simulink model "FOC_IF"  (R2023b)
settings: Solver=FixedStepDiscrete  StartTime=0.0  StopTime=1  FixedStep=0.000001  RelTol=1e-3
undefined symbols (not defined in the file): Pn, Udc
libraries: mcbplantlib x1, autolibpmsmexterior x1, simulink x1
settings Model: DataDictionary=SVPWM.sldd  Creator=18575  LastModifiedBy=Administrator

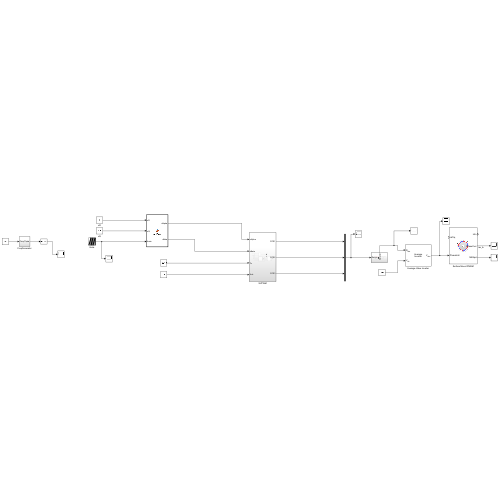
[thumbnail: Simulink's stored preview of the top-level diagram]
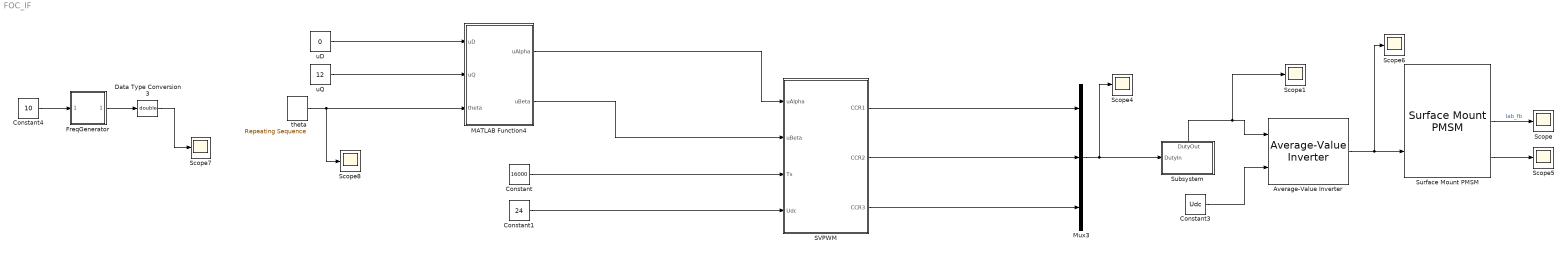
== system FOC_IF ==
  Average-Value Inverter : mcbplantlib/Average-Value Inverter
  Constant : Constant  Value=16000
  Constant1 : Constant  Value=24
  Constant3 : Constant  Value=Udc
  Constant4 : Constant  Value=10  OutDataTypeStr=single
  Data Type Conversion3 : DataTypeConversion  OutDataTypeStr=double  SaturateOnIntegerOverflow=off  RndMeth=Floor
  FreqGenerator : Subsystem
  MATLAB Function4 : MATLAB Function  TreatAsAtomicUnit=on
  Mux3 : Mux  Inputs=3
  SVPWM : Subsystem
  Scope{,1,4..8} (7 alike) : Scope
  Subsystem : Subsystem
      settings: PortSchema="{\"entries\":[{\"content\":{\"sides\":[{\"content\":{\"connectorIds\":[\"In1\"]},\"type\":\"ConnectorPlacement.EquallySpacedRectSide\",\"uuid\":\"8ccc51de-fa2a-4900-80a3-4cdf9aa76f01\"},{\"content\":{\"side\":\"RIGHT\"},\"type\":\"ConnectorPlacement.EquallySpacedRectSide\",\"uuid\":\"32c06e0d-3f1d-4948-af96-e310e54308a0\"},{\"content\":{\"connectorIds\":[\"Out1\"],\"side\":\"TOP\"},\"type\":\"ConnectorPlacement.EquallySpacedRectSide\",\"uuid\":\"a9066067-2c54-42a8-b4d7-fb86ac71b860\"}]},\"type\":\"ConnectorPlacement.EquallySpacedConnector\",\"uuid\":\"e4576975-acad-4e16-822f-2c2e7f23d7a7\"}],\"packageUris\":[\"http://schema.mathworks.com/mf0/Connector/R2020b\"],\"version\":\"1.0\"}"
  Surface Mount PMSM : autolibpmsmexterior/Surface Mount PMSM  port_config=Torque  sim_type=Discrete  Ts=1e-4  P=Pn  Rs=Rs  Ldq_=L  KConstText=Permanent flux linkage constant (lambda_pm):  lambda_pm=flux  Ke=0.0059268  Kt=0.061  mechanical=[75e-6, 8e-5, 0]  idq0=[0 0]  theta_init=4/5  omega_init=0  KConst=flux  lambda_pm_calc=flux  RefBlkName='autolibpmsmexterior/Surface Mount PMSM'  aMode=5  Ldq="[0.0017      0.0017]"
  "theta " : simulink/Sources/Repeating Sequence  rep_seq_t=[0 0.5]  rep_seq_y=[0 2*pi]
  uD : Constant  Value=0
  uQ : Constant  Value=12
  wires:
  uQ/1 -> MATLAB Function4/2(uQ)
  uD/1 -> MATLAB Function4/1(uD)
  Mux3/1 -> Scope4/1, Subsystem/1(DutyIn)
  Subsystem/1(DutyOut) -> Scope1/1, Average-Value Inverter/1
  Constant3/1 -> Average-Value Inverter/2
  Average-Value Inverter/1 -> Scope6/1, Surface Mount PMSM/2
  Surface Mount PMSM/2 -> Scope/1  "Iab_fb"
  Surface Mount PMSM/3 -> Scope5/1
  FreqGenerator/1(Theta) -> Data Type Conversion3/1
  Constant4/1 -> FreqGenerator/1(Freq)
  Data Type Conversion3/1 -> Scope7/1
  "theta "/1 -> Scope8/1, MATLAB Function4/3(theta)
  MATLAB Function4/1(uAlpha) -> SVPWM/1(uAlpha)
  MATLAB Function4/2(uBeta) -> SVPWM/2(uBeta)
  Constant/1 -> SVPWM/3(Ts)
  Constant1/1 -> SVPWM/4(Udc)
  SVPWM/1(CCR1) -> Mux3/1
  SVPWM/2(CCR2) -> Mux3/2
  SVPWM/3(CCR3) -> Mux3/3

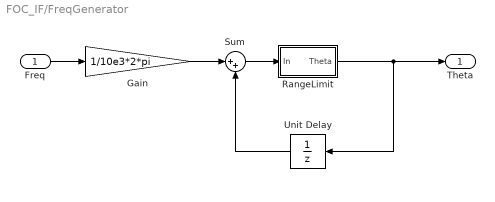
== system FOC_IF/FreqGenerator ==
  Freq : Inport
  Gain : Gain  Gain=1/10e3*2*pi  OutDataTypeStr=single
  RangeLimit : Subsystem
  Sum : Sum  Inputs=|++  OutDataTypeStr=Inherit: Same as first input
  Unit Delay : UnitDelay  SampleTime=-1  HasFrameUpgradeWarning=on
  Theta : Outport
  wires:
  Freq/1 -> Gain/1
  RangeLimit/1(Theta) -> Theta/1, Unit Delay/1
  Gain/1 -> Sum/1
  Sum/1 -> RangeLimit/1(In)
  Unit Delay/1 -> Sum/2

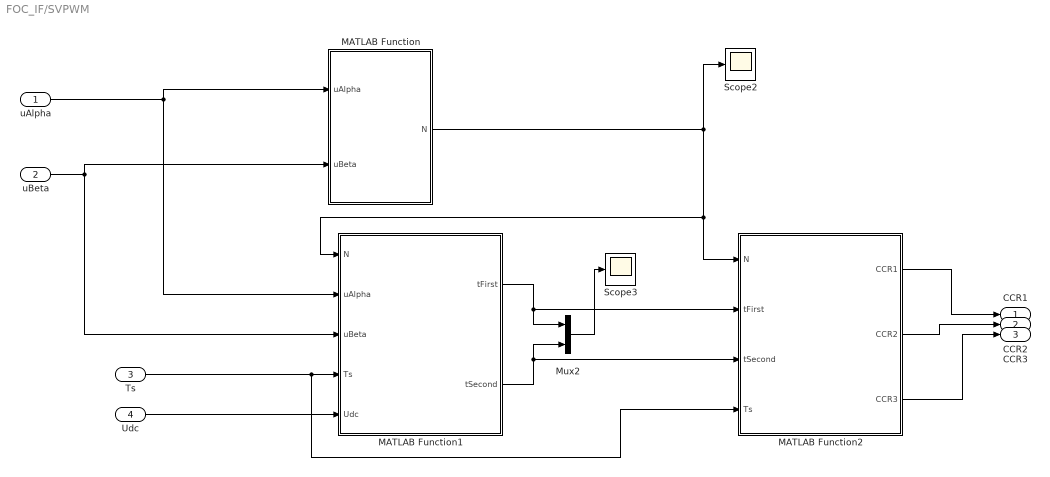
== system FOC_IF/SVPWM ==
  uAlpha : Inport
  uBeta : Inport  Port=2
  Ts : Inport  Port=3
  Udc : Inport  Port=4
  MATLAB Function : MATLAB Function  TreatAsAtomicUnit=on
  MATLAB Function1 : MATLAB Function  TreatAsAtomicUnit=on
  MATLAB Function2 : MATLAB Function  TreatAsAtomicUnit=on
  Mux2 : Mux  Inputs=2
  Scope2 : Scope
  Scope3 : Scope
  CCR1 : Outport
  CCR2 : Outport  Port=2
  CCR3 : Outport  Port=3
  wires:
  MATLAB Function2/2(CCR2) -> CCR2/1
  MATLAB Function/1(N) -> Scope2/1, MATLAB Function1/1(N), MATLAB Function2/1(N)
  MATLAB Function1/2(tSecond) -> MATLAB Function2/3(tSecond), Mux2/2
  MATLAB Function1/1(tFirst) -> MATLAB Function2/2(tFirst), Mux2/1
  Ts/1 -> MATLAB Function2/4(Ts), MATLAB Function1/4(Ts)
  uAlpha/1 -> MATLAB Function1/2(uAlpha), MATLAB Function/1(uAlpha)
  uBeta/1 -> MATLAB Function1/3(uBeta), MATLAB Function/2(uBeta)
  Mux2/1 -> Scope3/1
  MATLAB Function2/1(CCR1) -> CCR1/1
  MATLAB Function2/3(CCR3) -> CCR3/1
  Udc/1 -> MATLAB Function1/5(Udc)

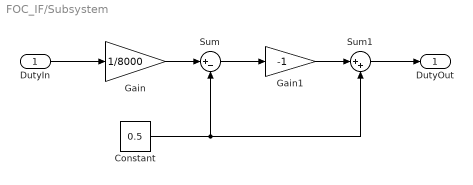
== system FOC_IF/Subsystem ==
  DutyIn : Inport
  Constant : Constant  Value=0.5  SampleTime=-1
  Gain : Gain  Gain=1/8000  ParamDataTypeStr=single
  Gain1 : Gain  Gain=-1
  Sum : Sum  Inputs=|+-
  Sum1 : Sum  Inputs=|++
  DutyOut : Outport
  wires:
  Sum/1 -> Gain1/1
  Constant/1 -> Sum1/2, Sum/2
  DutyIn/1 -> Gain/1
  Gain1/1 -> Sum1/1
  Sum1/1 -> DutyOut/1
  Gain/1 -> Sum/1

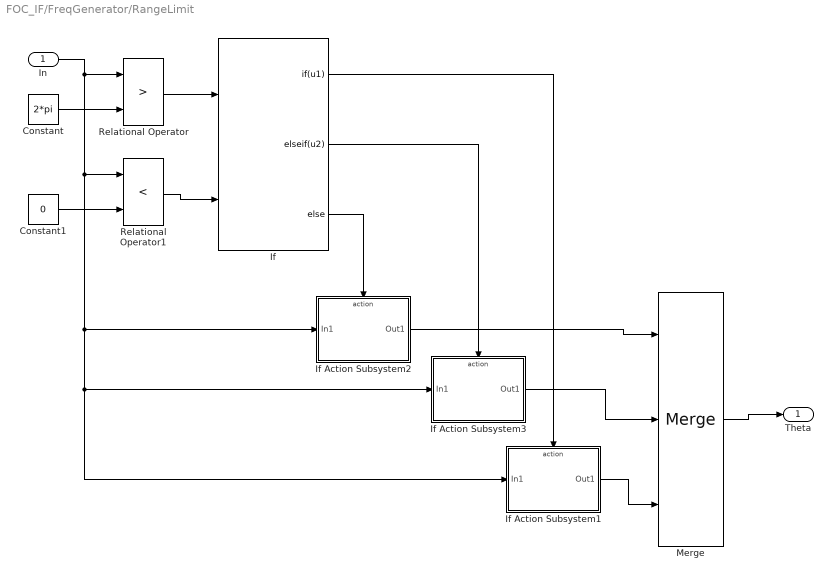
== system FOC_IF/FreqGenerator/RangeLimit ==
  In : Inport
  Constant : Constant  Value=2*pi  OutDataTypeStr=single  SampleTime=-1
  Constant1 : Constant  Value=0  OutDataTypeStr=single  SampleTime=-1
  If : If  NumInputs=2  IfExpression=u1  ElseIfExpressions=u2
  If Action Subsystem1 : Subsystem  TreatAsAtomicUnit=on
  If Action Subsystem2 : Subsystem  TreatAsAtomicUnit=on
  If Action Subsystem3 : Subsystem  TreatAsAtomicUnit=on
  Merge : Merge  Inputs=3
  Relational Operator : RelationalOperator  Operator=>  OutDataTypeStr=boolean  RndMeth=Simplest  InputSameDT=off
  Relational Operator1 : RelationalOperator  Operator=<  OutDataTypeStr=boolean  RndMeth=Simplest  InputSameDT=off
  Theta : Outport
  wires:
  Relational Operator/1 -> If/1
  Constant/1 -> Relational Operator/2
  In/1 -> Relational Operator1/1, If Action Subsystem2/1(In1), If Action Subsystem3/1(In1), If Action Subsystem1/1(In1), Relational Operator/1
  Merge/1 -> Theta/1
  If/3 -> If Action Subsystem2/Action
  If/1 -> If Action Subsystem1/Action
  If Action Subsystem2/1(Out1) -> Merge/1
  Constant1/1 -> Relational Operator1/2
  Relational Operator1/1 -> If/2
  If/2 -> If Action Subsystem3/Action
  If Action Subsystem1/1(Out1) -> Merge/3
  If Action Subsystem3/1(Out1) -> Merge/2

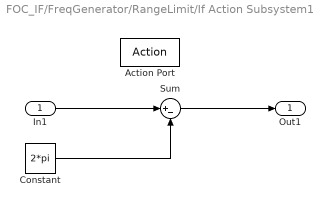
== system FOC_IF/FreqGenerator/RangeLimit/If Action Subsystem1 ==
  In1 : Inport
  Action Port : ActionPort  ActionPortLabel=if(u1)
  Constant : Constant  Value=2*pi  OutDataTypeStr=single  SampleTime=-1
  Sum : Sum  Inputs=|+-
  Out1 : Outport
  wires:
  In1/1 -> Sum/1
  Constant/1 -> Sum/2
  Sum/1 -> Out1/1

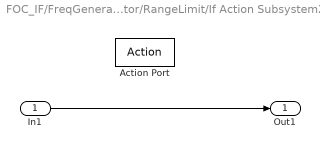
== system FOC_IF/FreqGenerator/RangeLimit/If Action Subsystem2 ==
  In1 : Inport
  Action Port : ActionPort  ActionPortLabel=else
  Out1 : Outport
  wires:
  In1/1 -> Out1/1

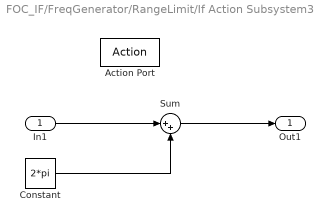
== system FOC_IF/FreqGenerator/RangeLimit/If Action Subsystem3 ==
  In1 : Inport
  Action Port : ActionPort  ActionPortLabel=elseif(u2)
  Constant : Constant  Value=2*pi  OutDataTypeStr=single  SampleTime=-1
  Sum : Sum  Inputs=|++
  Out1 : Outport
  wires:
  Constant/1 -> Sum/2
  In1/1 -> Sum/1
  Sum/1 -> Out1/1

== matlab function FOC_IF/SVPWM/MATLAB Function1 ==
  data: N input; tFirst output; uAlpha input; uBeta input; tSecond output; Ts input; Udc input
function [tFirst, tSecond] = vectorCalculate(N, uAlpha, uBeta, Ts, Udc)

tFirst = 0;
tSecond = 0;

X = sqrt(3)*Ts*uBeta/Udc;
Y = sqrt(3)*Ts/Udc*(sqrt(3)*uAlpha/2+uBeta/2);
Z = sqrt(3)*Ts/Udc*(-sqrt(3)*uAlpha/2+uBeta/2);

if (N == 1)
    tFirst = Z;
    tSecond = Y;
end

if (N==2)
    tFirst = Y;
    tSecond = -X;
end

if (N==3)
    tFirst =-Z;
    tSecond = X;
end

if (N==4)
    tFirst =-X;
    tSecond = Z;
end

if (N==5)
    tFirst =X;
    tSecond = -Y;
end

if (N==6)
    tFirst =-Y;
    tSecond = -Z;
end

== matlab function FOC_IF/SVPWM/MATLAB Function ==
  data: uAlpha input; N output; uBeta input

function N = sectorJudge(uAlpha, uBeta)

u1 = uBeta;
u2 = sqrt(3)/2*uAlpha - 1/2*uBeta;
u3 = -sqrt(3)/2*uAlpha - 1/2*uBeta;

N = 0;
if (u1 > 0)
    N = N+1;
end;

if (u2 > 0)
    N = N+2;
end;

if (u3 > 0)
    N = N+4;
end;

== matlab function FOC_IF/SVPWM/MATLAB Function2 ==
  data: N input; CCR1 output; tFirst input; tSecond input; CCR2 output; Ts input; CCR3 output
function [CCR1, CCR2, CCR3] =  CCR_calculate(N, tFirst, tSecond,  Ts)

CCR1 = 0;
CCR2 = 0;
CCR3 = 0;

t = tFirst + tSecond;
if (t > Ts)
    tFirst = tFirst/t * Ts;
    tSecond = tSecond / t * Ts;
end

value1 = (Ts - tFirst - tSecond) /4;  % vector 0 or 7 
value2 = value1 + tFirst / 2;
value3 = value2 + tSecond / 2;

switch(N)
    case 3
        CCR1 = value1;
        CCR2 = value2;
        CCR3 = value3;

    case 1
        CCR1 = value2;
        CCR2 = value1;
        CCR3 = value3;

    case 5
        CCR1 = value3;
        CCR2 = value1;
        CCR3 = value2;

    case 4
        CCR1 = value3;
        CCR2 = value2;
        CCR3 = value1;

    case 6
        CCR1 = value2;
        CCR2 = value3;
        CCR3 = value1;

    case 2
        CCR1 = value1;
        CCR2 = value3;
        CCR3 = value2;

end

== matlab function FOC_IF/MATLAB Function4 ==
  data: uD input; uAlpha output; uQ input; theta input; uBeta output
function [uAlpha, uBeta] = revPark(uD, uQ, theta)


uAlpha = 0;
uBeta = 0;

uAlpha = cos(theta) * uD - sin(theta) *uQ;
uBeta = sin(theta) * uD + cos(theta) * uQ;
